simulink model "Sim_Ob_Edo (1)"  (R2021b)
settings: Solver=VariableStepAuto  StartTime=0.0  StopTime=20  RelTol=1e-3  EnableMultiTasking=on
values from neighbouring files (symbols this model uses):
  A = [-a1 1 0;-a2 0 1;-a3 0 0]    [Ob_EdoEx.m]    (also in examen.m = Acc)
  Ak = A + k*c.'    [Ob_EdoEx.m]    (also in examen.m = A + k'*c.')
  b = [0;0;1]    [Ob_EdoEx.m]    (also in examen.m = bcc)
  Id = eye(3)    [Ob_EdoEx.m]    (also in examen.m)
  k = T1*ko    [Ob_EdoEx.m]    (also in examen.m = kcc)
  vcero = zeros(3,1)    [Ob_EdoEx.m]    (also in examen.m)
  x0 = [-1; 0; 0]    [Ob_EdoEx.m]    (also in examen.m = [-1;0;0])
undefined symbols (not defined in the file or in its folder): T2
settings Model: Creator=Tlayekanketl  LastModifiedBy=Idael
settings SolverCC: AlgebraicLoopSolver=TrustRegion
settings DataIOCC: LimitDataPoints=on  SaveFormat=Array  SignalLoggingSaveFormat=ModelDataLogs  ReturnWorkspaceOutputs=off
settings OptimizationCC: ExpressionDepthLimit=2147483647  LifeSpan=inf
settings DebuggingCC: UnderspecifiedInitializationDetection=Classic  MergeDetectMultiDrivingBlocksExec=none  FcnCallInpInsideContextMsg=warning  AllowSymbolicDim=off  StateNameClashWarn=warning  SFUnexpectedBacktrackingDiag=warning  SFNoUnconditionalDefaultTransitionDiag=warning  SFExecutionAtInitializationDiag=none  SFMachineParentedDataDiag=warning  ArithmeticOperatorsInVariantConditions=warning
settings HardwareCC: ProdBitPerPointer=32  ProdBitPerSizeT=32  ProdBitPerPtrDiffT=32  ProdLargestAtomicFloat=None  ProdIntDivRoundTo=Undefined  ProdEndianess=Unspecified  ProdWordSize=32  ProdHWDeviceType=32-bit Generic
settings ModelReferenceCC: PropagateSignalLabelsOutOfModel=off
settings SFSimCC: SimUseLocalCustomCode=off  CustomCodeUndefinedFunction=UseInterfaceOnly
settings RTWCC: RTWUseLocalCustomCode=off
settings CodeAppCC: StateflowObjectComments=on
settings GRTTargetCC: TargetLangStandard=C89/C90 (ANSI)  CombineOutputUpdateFcns=off  GRTInterface=on
settings ConfigComp: CovMetricSettings=dw  CovSaveCumulativeToWorkspaceVar=on  CovSaveSingleToWorkspaceVar=on  CovExternalEMLEnable=off  CovSFcnEnable=off

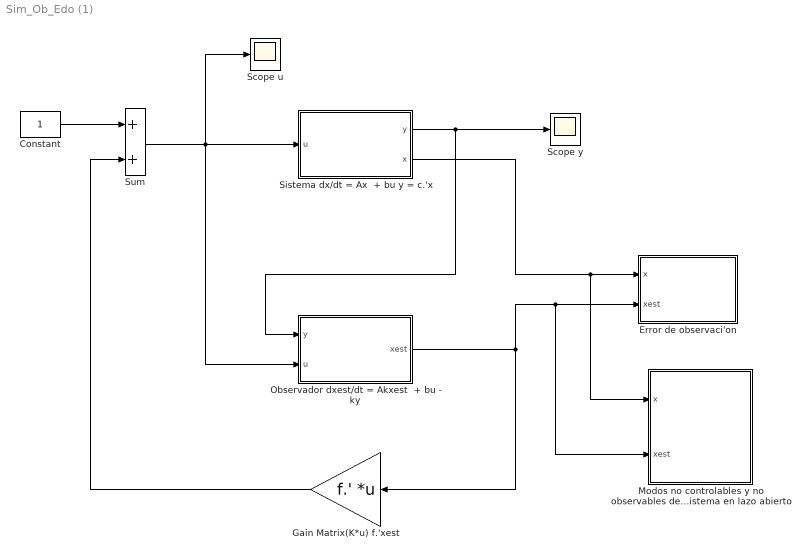
== system Sim_Ob_Edo (1) ==
  Constant : Constant
  Error de observaci'on : Subsystem
  Gain Matrix(K*u) f.'xest : Gain  Gain=f.'  Multiplication=Matrix(K*u) (u vector)
  Modos no controlables y no observables del sistema en lazo abierto : Subsystem
  Observador dxest/dt = Akxest  + bu - ky : Subsystem
  Scope u : Scope
  Scope y : Scope
  Sistema dx/dt = Ax  + bu y = c.'x : Subsystem
  Sum : Sum
  wires:
  Sum/1 -> Sistema dx/dt = Ax  + bu y = c.'x/1(u), Observador dxest/dt = Akxest  + bu - ky/2(u), Scope u/1
  Constant/1 -> Sum/1
  Gain Matrix(K*u) f.'xest/1 -> Sum/2
  Observador dxest/dt = Akxest  + bu - ky/1(xest) -> Gain Matrix(K*u) f.'xest/1, Error de observaci'on/2(xest), Modos no controlables y no observables del sistema en lazo abierto/2(xest)
  Sistema dx/dt = Ax  + bu y = c.'x/1(y) -> Scope y/1, Observador dxest/dt = Akxest  + bu - ky/1(y)
  Sistema dx/dt = Ax  + bu y = c.'x/2(x) -> Error de observaci'on/1(x), Modos no controlables y no observables del sistema en lazo abierto/1(x)

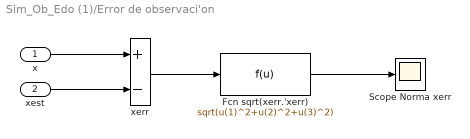
== system Sim_Ob_Edo (1)/Error de observaci'on ==
  x : Inport
  xest : Inport  Port=2
  Fcn sqrt(xerr.'xerr) : Fcn  Expr=sqrt(u(1)^2+u(2)^2+u(3)^2)
  Scope Norma xerr : Scope
  xerr : Sum  Inputs=+-
  wires:
  xerr/1 -> Fcn sqrt(xerr.'xerr)/1
  Fcn sqrt(xerr.'xerr)/1 -> Scope Norma xerr/1
  xest/1 -> xerr/2
  x/1 -> xerr/1

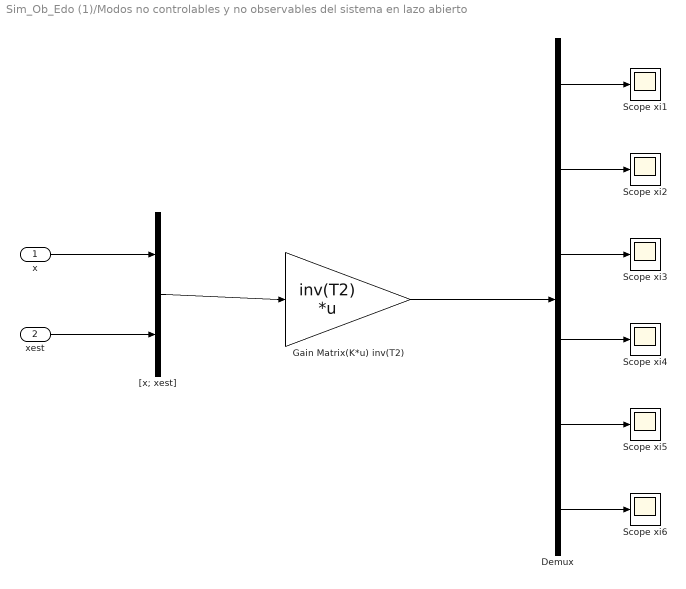
== system Sim_Ob_Edo (1)/Modos no controlables y no observables del sistema en lazo abierto ==
  x : Inport
  xest : Inport  Port=2
  Demux : Demux  Outputs=6
  Gain Matrix(K*u) inv(T2) : Gain  Gain=inv(T2)  Multiplication=Matrix(K*u) (u vector)
  Scope xi{1..6} (6 alike) : Scope
  "[x; xest]" : Mux  Inputs=2
  wires:
  x/1 -> "[x; xest]"/1
  xest/1 -> "[x; xest]"/2
  "[x; xest]"/1 -> Gain Matrix(K*u) inv(T2)/1
  Demux/3 -> Scope xi3/1
  Demux/2 -> Scope xi2/1
  Demux/1 -> Scope xi1/1
  Demux/4 -> Scope xi4/1
  Demux/5 -> Scope xi5/1
  Demux/6 -> Scope xi6/1
  Gain Matrix(K*u) inv(T2)/1 -> Demux/1

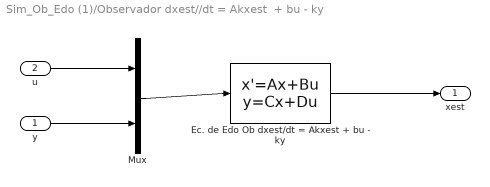
== system Sim_Ob_Edo (1)/Observador dxest//dt = Akxest  + bu - ky ==
  y : Inport
  u : Inport  Port=2
  Ec. de Edo Ob dxest/dt = Akxest + bu - ky : StateSpace  A=Ak  B=[b -k]  C=Id  D=[vcero vcero]  InitialCondition=vcero
  Mux : Mux  Inputs=2
  xest : Outport
  wires:
  Mux/1 -> Ec. de Edo Ob dxest/dt = Akxest + bu - ky/1
  Ec. de Edo Ob dxest/dt = Akxest + bu - ky/1 -> xest/1
  u/1 -> Mux/1
  y/1 -> Mux/2

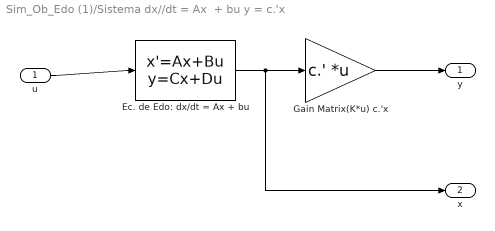
== system Sim_Ob_Edo (1)/Sistema dx//dt = Ax  + bu y = c.'x ==
  u : Inport
  Ec. de Edo: dx/dt = Ax + bu : StateSpace  A=A  B=b  C=Id  D=vcero  InitialCondition=x0
  Gain Matrix(K*u) c.'x : Gain  Gain=c.'  Multiplication=Matrix(K*u) (u vector)
  y : Outport
  x : Outport  Port=2
  wires:
  u/1 -> Ec. de Edo: dx/dt = Ax + bu/1
  Ec. de Edo: dx/dt = Ax + bu/1 -> Gain Matrix(K*u) c.'x/1, x/1
  Gain Matrix(K*u) c.'x/1 -> y/1
